simulink model "Elevation_system"  (R2022b)
settings: Solver=VariableStepAuto  StartTime=0.0  StopTime=10  RelTol=1e-4
undefined symbols (not defined in the file): C_pi_pod_elev, C_pi_pod_elev_Kp, gain_notch_pod_elev_tf, k_egun_inv_plant, k_feed_gun_elev, linear_egun_inv_plant, linear_feed_forward_GUN_elev_dist
libraries: slpidlib x2, simulink x1
settings Model: Creator=ohadformanair  LastModifiedBy=ohadformanair
settings SolverCC: ZeroCrossAlgorithm=Adaptive
settings DebuggingCC: MaskedZcDiagnostic=none  IgnoredZcDiagnostic=none
settings ModelReferenceCC: EnableRefExpFcnMdlSchedulingChecks=on

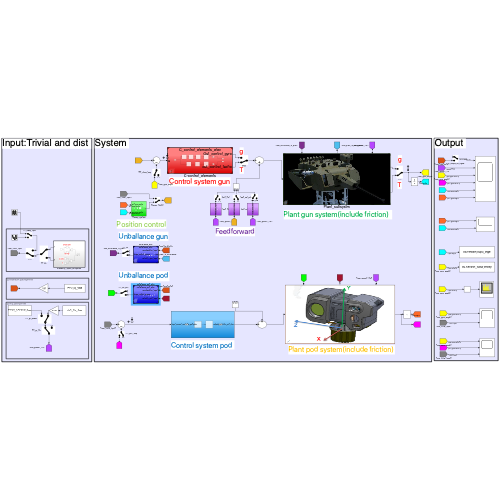
[thumbnail: Simulink's stored preview of the top-level diagram]
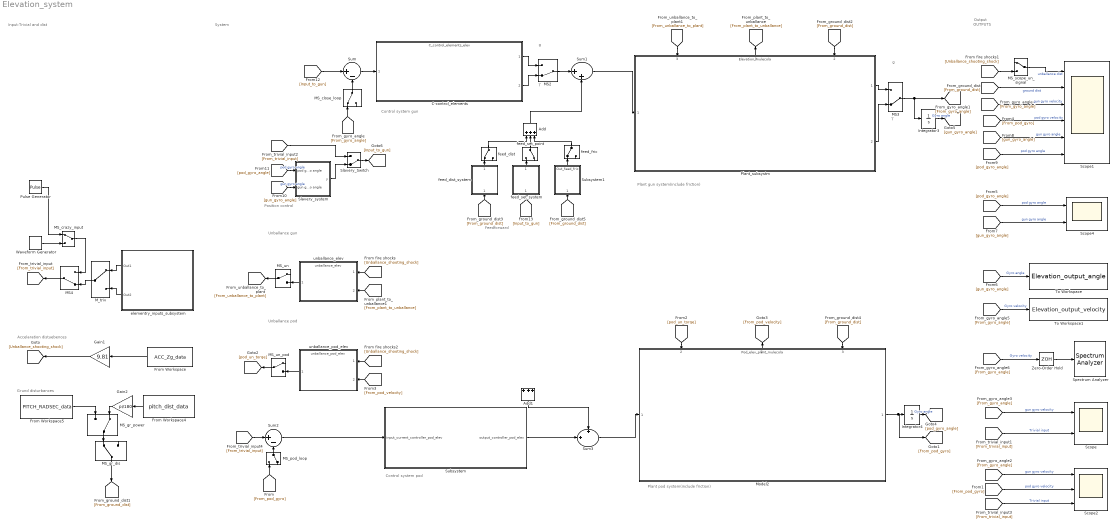
== system Elevation_system ==
  note: Input:Trivial and dist
  note: Control system gun
  note: Accelaration distuebences
  note: Grund disturbances
  note: OUTPUTS
  note: T
  note: T
  note: g
  note: g
  note: Plant gun system(include friction)
  note: Unballance gun
  note: System
  note: Output
  note: Feedforward
  note: Plant pod system(include friction)
  note: Control system pod
  note: Unballance pod
  note: Position control
  Add : Sum  Inputs=+++
  Add1 : Sum  Inputs=+++
  C-control_elements : ModelReference  ModelNameDialog=C_control_elements_elev  SimulationMode=Normal  ModelReferenceVersion=2.0
  From Workspace : FromWorkspace  VariableName=ACC_Zg_data  SampleTime=-1
  From Workspace4 : FromWorkspace  VariableName=pitch_dist_data  SampleTime=-1
  From Workspace5 : FromWorkspace  VariableName=PITCH_RADSEC_data  SampleTime=-1
  Gain1 : Gain  Gain=9.81
  Gain2 : Gain  Gain=pi/180
  Integrator3 : Integrator
  Integrator4 : Integrator
  MS2 : ManualSwitch  CurrentSetting=0
  MS3 : ManualSwitch  CurrentSetting=0
  MS4 : ManualSwitch  CurrentSetting=0
  MS_close_loop : ManualSwitch
  MS_crazy_input : ManualSwitch
  MS_gr_dis : ManualSwitch
  MS_gr_power : ManualSwitch  CurrentSetting=0
  MS_pod_loop : ManualSwitch  CurrentSetting=0
  MS_scope_un_signal : ManualSwitch
  MS_un : ManualSwitch
  MS_un_pod : ManualSwitch
  M_triv : ManualSwitch
  Model2 : ModelReference  ModelNameDialog=Pod_elev_plant_mulecola  SimulationMode=Normal  ModelReferenceVersion=1.13
      settings: PortSchema="{\"entries\":[{\"content\":{\"sides\":[{\"content\":{\"connectorIds\":[\"In1\"]},\"type\":\"ConnectorPlacement.EquallySpacedRectSide\",\"uuid\":\"9e025463-df89-4145-8e3a-d977ce9d23dd\"},{\"content\":{\"connectorIds\":[\"Out1\"],\"side\":\"RIGHT\"},\"type\":\"ConnectorPlacement.EquallySpacedRectSide\",\"uuid\":\"8c795400-902a-445d-a152-b91382759f27\"},{\"content\":{\"connectorIds\":[\"In2\",\"Out2\",\"In3\"],\"side\":\"TOP\"},\"type\":\"ConnectorPlacement.EquallySpacedRectSide\",\"uuid\":\"4797fa26-c9ab-404f-8ecb-3633ee4e5d95\"}]},\"type\":\"ConnectorPlacement.EquallySpacedConnector\",\"uuid\":\"8bb34f86-ba6d-4f3e-a062-415220e2f7a6\"}],\"packageUris\":[\"http://schema.mathworks.com/mf0/Connector/R2020b\"],\"version\":\"1.0\"}"
      mask Display: image('/Users/ohadformanair/Desktop/צילום מסך 2022-12-07 ב-4.14.47.png'); % Use "Edit Image" on toolstrip to change.
  Plant_subsystm : ModelReference  ModelNameDialog=Elevation_mulecola.slx  SimulationMode=Normal  ModelReferenceVersion=2.22
      settings: PortSchema="{\"entries\":[{\"content\":{\"sides\":[{\"content\":{\"connectorIds\":[\"In1\"]},\"type\":\"ConnectorPlacement.EquallySpacedRectSide\",\"uuid\":\"5c3be150-06c1-4b04-81d4-c89054a50b58\"},{\"content\":{\"connectorIds\":[\"Out1\",\"Out2\"],\"side\":\"RIGHT\"},\"type\":\"ConnectorPlacement.EquallySpacedRectSide\",\"uuid\":\"5dfcaa34-ef70-477d-9189-6856ebc4bbcf\"},{\"content\":{\"connectorIds\":[\"In3\",\"Out3\",\"In2\"],\"side\":\"TOP\"},\"type\":\"ConnectorPlacement.EquallySpacedRectSide\",\"uuid\":\"06d3d264-a507-4be0-8bff-1d5586be5fcb\"},{\"content\":{\"connectorIds\":[],\"side\":\"BOTTOM\"},\"type\":\"ConnectorPlacement.EquallySpacedRectSide\",\"uuid\":\"978608b5-cbbf-4f72-8870-46e3c0d8a99d\"}]},\"type\":\"ConnectorPlacement.EquallySpacedConnector\",\"uuid\":\"1f4e30e1-d134-49fc-8bd6-0842cd83f06c\"}],\"packageUris\":[\"http://schema.mathworks.com/mf0/Connector/R2020b\"],\"version\":\"1.0\"}"
      mask Display: image('/Users/ohadformanair/Desktop/צילום מסך 2022-12-07 ב-4.16.46.png'); % Use "Edit Image" on toolstrip to change.
  Pulse Generator : DiscretePulseGenerator  PulseType=Time based  Period=1  PulseWidth=50
  Scope : Scope  NumInputPorts=2
  Scope1 : Scope  NumInputPorts=6
  Scope2 : Scope  NumInputPorts=3
  Scope4 : Scope  NumInputPorts=2
  Slavery_Switch : ManualSwitch  CurrentSetting=0
  Slavery_system : Subsystem
  Spectrum Analyzer : SpectrumAnalyzer
  Subsystem : Subsystem
  Subsystem1 : Subsystem
  Sum : Sum  Inputs=|+-
  Sum1 : Sum  Inputs=|++
  Sum2 : Sum  Inputs=|+-
  Sum3 : Sum  Inputs=+|+||
  To Workspace : ToWorkspace  VariableName=Elevation_output_angle  SaveFormat=Timeseries  SampleTime=-1
  To Workspace1 : ToWorkspace  VariableName=Elevation_output_velocity  SaveFormat=Timeseries  SampleTime=-1
  Waveform Generator : simulink/Sources/Waveform Generator  OutMin=[]  OutMax=[]  OutDataTypeStr=double  SelectedSignal=1  Signals=sin(sawtooth(1,2,0),1,2)+Square(1,2,0,50)#Square(1,2,0,50)  BlockNames=MultiportSwitch_bb3116ca3c8c4cb#MultiportSwitch_6d83ebdfd0d2480  SampleTime=0.01
  Zero-Order Hold : ZeroOrderHold  SampleTime=0.001
  elementry_inputs_subsystem : Subsystem  TreatAsAtomicUnit=on
  feed_dist : ManualSwitch
  feed_dist_system : Subsystem
  feed_fric : ManualSwitch
  feed_set_point : ManualSwitch  CurrentSetting=0
  feed_set_system : Subsystem
  unballance_elev : ModelReference  ModelNameDialog=unballance_elev.slx  SimulationMode=Normal  ModelReferenceVersion=1.10
  unballance_pod_elev : ModelReference  ModelNameDialog=unballance_pod_elev.slx  SimulationMode=Normal  ModelReferenceVersion=1.12
  wires:
  MS_close_loop/1 -> Sum/2
  Plant_subsystm/2 -> MS3/2
  M_triv/1 -> MS4/2
  From Workspace5/1 -> MS_gr_power/1
  MS_gr_power/1 -> MS_gr_dis/1
  [gun_gyro_angle] -> To Workspace/1  "Gyro angle"
  From Workspace4/1 -> Gain2/1
  Gain2/1 -> MS_gr_power/2
  C-control_elements/2 -> MS2/2
  elementry_inputs_subsystem/1(Out1) -> M_triv/1
  elementry_inputs_subsystem/2(Out2) -> M_triv/2
  unballance_elev/1 -> MS_un/2
  Gain1/1 -> [Unballance_shooting_shock]
  C-control_elements/1 -> MS2/1
  Plant_subsystm/1 -> MS3/1
  From Workspace/1 -> Gain1/1
  Sum/1 -> C-control_elements/1
  Zero-Order Hold/1 -> Spectrum Analyzer/1
  MS_scope_un_signal/1 -> Scope1/1  "unballance dist"
  MS2/1 -> Sum1/1
  [Unballance_shooting_shock] -> unballance_elev/1
  [Unballance_shooting_shock] -> MS_scope_un_signal/2
  MS_gr_dis/1 -> [From_ground_dist]
  [From_ground_dist] -> Plant_subsystm/2
  MS3/1 -> [From_gyro_angle], Integrator3/1
  [From_gyro_angle] -> MS_close_loop/1
  [From_trivial_input] -> Slavery_Switch/1
  MS4/1 -> [From_trivial_input]
  Plant_subsystm/3 -> [From_plant_to_unballance]
  [From_plant_to_unballance] -> unballance_elev/2
  MS_un/1 -> [From_unballance_to_plant]
  [From_unballance_to_plant] -> Plant_subsystm/3
  [From_ground_dist] -> Scope1/2  "ground dist"
  Sum1/1 -> Plant_subsystm/1
  Sum2/1 -> Subsystem/1(input_current_controller_pod_elev)
  [From_trivial_input] -> Sum2/1
  MS_pod_loop/1 -> Sum2/2
  Model2/1 -> [From_pod_gyro], Integrator4/1
  Add/1 -> Sum1/2
  feed_dist/1 -> Add/1
  feed_set_point/1 -> Add/2
  [From_ground_dist] -> feed_dist_system/1(feed_dist_input)
  feed_dist_system/1(feed_dist_output) -> feed_dist/1
  feed_set_system/1(feed_set_output) -> feed_set_point/1
  [Input_to_gun] -> feed_set_system/1(feed_set_input)
  [From_trivial_input] -> Scope/2  "Trivial input"
  MS_crazy_input/1 -> MS4/1
  Waveform Generator/1 -> MS_crazy_input/2
  [From_pod_gyro] -> MS_pod_loop/1
  [From_pod_gyro] -> Scope2/2  "pod gyro velocity"
  [From_trivial_input] -> Scope2/3  "Trivial input"
  [From_pod_velocity] -> unballance_pod_elev/2
  Model2/2 -> [From_pod_velocity]
  [Unballance_shooting_shock] -> unballance_pod_elev/1
  unballance_pod_elev/1 -> MS_un_pod/2
  MS_un_pod/1 -> [pod_un_torqe]
  [pod_un_torqe] -> Model2/2
  [From_ground_dist] -> Model2/3
  Subsystem/1(output_controller_pod_elev) -> Sum3/2
  Sum3/1 -> Model2/1
  [From_pod_gyro] -> Scope1/4  "pod gyro velocity"
  [From_gyro_angle] -> Scope2/1  "gun gyro velocity"
  feed_fric/1 -> Add/3
  [From_ground_dist] -> Subsystem1/1(In_dist_velocity)
  Subsystem1/1(Out_feed_fric) -> feed_fric/1
  Integrator3/1 -> [gun_gyro_angle]  "Gyro angle"
  Integrator4/1 -> [pod_gyro_angle]  "Gyro angle"
  [pod_gyro_angle] -> Scope4/1  "pod gyro angle"
  [gun_gyro_angle] -> Scope4/2  "gun gyro angle"
  [gun_gyro_angle] -> Scope1/5  "gun gyro angle"
  [From_gyro_angle] -> Scope/1  "gun gyro velocity"
  [From_gyro_angle] -> To Workspace1/1  "Gyro velocity"
  [From_gyro_angle] -> Scope1/3  "gun gyro velocity"
  [pod_gyro_angle] -> Scope1/6  "pod gyro angle"
  [From_gyro_angle] -> Zero-Order Hold/1  "Gyro velocity"
  Add1/1 -> Sum3/1
  Slavery_Switch/1 -> [Input_to_gun]
  [pod_gyro_angle] -> Slavery_system/1(pod gyro angle)  "pod gyro angle"
  [gun_gyro_angle] -> Slavery_system/2(gun gyro angle)  "gun gyro angle"
  Slavery_system/1(y) -> Slavery_Switch/2
  [Input_to_gun] -> Sum/1
  Pulse Generator/1 -> MS_crazy_input/1

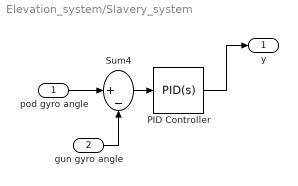
== system Elevation_system/Slavery_system ==
  pod gyro angle : Inport
  gun gyro angle : Inport  Port=2
  PID Controller : slpidlib/PID Controller  Controller=PID  Form=Parallel  TimeDomain=Continuous-time  UseExternalTs=off  SampleTime=-1  IntegratorMethod=Forward Euler  FilterMethod=Forward Euler  ControllerParametersSource=internal  P=28.4604839223426+30  I=9.47112032466826  UseKiTs=off  D=0.287192930745774  N=4361.00624343209  UseFilter=on  TunerSelectOption=Transfer Function Based (PID Tuner App)  InitialConditionSource=internal  InitialConditionForIntegrator=0  InitialConditionForFilter=0  DifferentiatorICPrevScaledInput=0  ExternalReset=none  TrackingMode=off  Kt=1  LimitOutput=off  SatLimitsSource=internal  UpperSaturationLimit=inf  LowerSaturationLimit=-inf  LinearizeAsGain=on  AntiWindupMode=none  Kb=1  LimitIntegrator=off  UpperIntegratorSaturationLimit=inf  LowerIntegratorSaturationLimit=-inf  POutMin=[]  POutMax=[]  IOutMin=[]  IOutMax=[]  DOutMin=[]  DOutMax=[]  NOutMin=[]  NOutMax=[]  SumOutMin=[]  SumOutMax=[]  SaturationOutMin=[]  SaturationOutMax=[]  PParamMin=[]  PParamMax=[]  IParamMin=[]  IParamMax=[]  DParamMin=[]  DParamMax=[]  NParamMin=[]  NParamMax=[]  KbParamMin=[]  KbParamMax=[]  KtParamMin=[]  KtParamMax=[]  KbOutMin=[]  KbOutMax=[]  KtOutMin=[]  KtOutMax=[]  IntegratorOutMin=[]  IntegratorOutMax=[]  FilterOutMin=[]  FilterOutMax=[]  SumI1OutMin=[]  SumI1OutMax=[]  SumI2OutMin=[]  SumI2OutMax=[]  SumI3OutMin=[]  SumI3OutMax=[]  SumI4OutMin=[]  SumI4OutMax=[]  SumDOutMin=[]  SumDOutMax=[]  DifferentiatorOutMin=[]  DifferentiatorOutMax=[]  FilterDiffOutCoefMin=[]  FilterDiffOutCoefMax=[]  ReciprocalOutMin=[]  ReciprocalOutMax=[]  SumDenOutMin=[]  SumDenOutMax=[]  SumNumOutMin=[]  SumNumOutMax=[]  DivideOutMin=[]  DivideOutMax=[]  UdiffTsProdOutMin=[]  UdiffTsProdOutMax=[]  NTsProdOutMin=[]  NTsProdOutMax=[]  UintegralTsProdOutMin=[]  UintegralTsProdOutMax=[]  UngainTsProdOutMin=[]  UngainTsProdOutMax=[]  ClampingZeroOutDataTypeStr=Inherit: Inherit via back propagation  ClampingZeroOutMin=[]  ClampingZeroOutMax=[]  FilterDenConstantOutDataTypeStr=Inherit: Inherit via back propagation  FilterDenConstantOutMin=[]  FilterDenConstantOutMax=[]  PCopyOutDataTypeStr=Inherit: Inherit via back propagation  PCopyOutMin=[]  PCopyOutMax=[]  NCopyOutDataTypeStr=Inherit: Inherit via back propagation  NCopyOutMin=[]  NCopyOutMax=[]  IntegratorContinuousStateAttributes=''  IntegratorStateMustResolveToSignalObject=off  IntegratorRTWStateStorageClass=Auto  FilterContinuousStateAttributes=''  FilterStateMustResolveToSignalObject=off  FilterRTWStateStorageClass=Auto  ParallelPVariant=InternalParameters  IdealPVariant=Disabled  IVariant=InternalParameters  DVariant=InternalParameters  IntegratorVariant=Continuous  SatVariant=Disabled  AWVariant=Passthrough  PCopyVariant=Disabled  TRVariant=Disabled  FdbkBlocksVariant=Forward  IdealPFdbkVariant=Disabled  SatFdbkVariant=Disabled  DerivativeFilterVariant=ContFilter  NVariant=InternalParameters  NCopyVariant=Disabled  FilterICVariant=InternalICsFilter  IntegratorICVariant=InternalICs  ExternalResetVariant=Disabled  TRSumVariant=Passthrough  SumFdbkVariant=Disabled  SumVariant=Sum_PID  TsampFilterVariant=InternalTs  TsampNgainVariant=Passthrough  TsampIntegralVariant=Passthrough  ExternalSaturationOutDataTypeStr=Inherit: Same as second input
  Sum4 : Sum  Inputs=|+-
  y : Outport
  wires:
  pod gyro angle/1 -> Sum4/1
  PID Controller/1 -> y/1
  gun gyro angle/1 -> Sum4/2
  Sum4/1 -> PID Controller/1

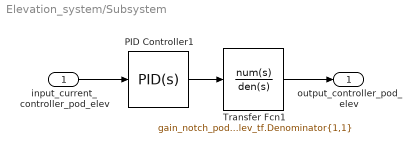
== system Elevation_system/Subsystem ==
  input_current_controller_pod_elev : Inport
  PID Controller1 : slpidlib/PID Controller  Controller=PID  Form=Parallel  TimeDomain=Continuous-time  UseExternalTs=off  SampleTime=-1  IntegratorMethod=Forward Euler  FilterMethod=Forward Euler  ControllerParametersSource=internal  P=C_pi_pod_elev_Kp  I=C_pi_pod_elev.Ki  UseKiTs=off  D=0  N=0  UseFilter=on  TunerSelectOption=Transfer Function Based (PID Tuner App)  InitialConditionSource=internal  InitialConditionForIntegrator=0  InitialConditionForFilter=0  DifferentiatorICPrevScaledInput=0  ExternalReset=none  TrackingMode=off  Kt=1  LimitOutput=off  SatLimitsSource=internal  UpperSaturationLimit=inf  LowerSaturationLimit=-inf  LinearizeAsGain=on  AntiWindupMode=none  Kb=1  LimitIntegrator=off  UpperIntegratorSaturationLimit=inf  LowerIntegratorSaturationLimit=-inf  POutMin=[]  POutMax=[]  IOutMin=[]  IOutMax=[]  DOutMin=[]  DOutMax=[]  NOutMin=[]  NOutMax=[]  SumOutMin=[]  SumOutMax=[]  SaturationOutMin=[]  SaturationOutMax=[]  PParamMin=[]  PParamMax=[]  IParamMin=[]  IParamMax=[]  DParamMin=[]  DParamMax=[]  NParamMin=[]  NParamMax=[]  KbParamMin=[]  KbParamMax=[]  KtParamMin=[]  KtParamMax=[]  KbOutMin=[]  KbOutMax=[]  KtOutMin=[]  KtOutMax=[]  IntegratorOutMin=[]  IntegratorOutMax=[]  FilterOutMin=[]  FilterOutMax=[]  SumI1OutMin=[]  SumI1OutMax=[]  SumI2OutMin=[]  SumI2OutMax=[]  SumI3OutMin=[]  SumI3OutMax=[]  SumI4OutMin=[]  SumI4OutMax=[]  SumDOutMin=[]  SumDOutMax=[]  DifferentiatorOutMin=[]  DifferentiatorOutMax=[]  FilterDiffOutCoefMin=[]  FilterDiffOutCoefMax=[]  ReciprocalOutMin=[]  ReciprocalOutMax=[]  SumDenOutMin=[]  SumDenOutMax=[]  SumNumOutMin=[]  SumNumOutMax=[]  DivideOutMin=[]  DivideOutMax=[]  UdiffTsProdOutMin=[]  UdiffTsProdOutMax=[]  NTsProdOutMin=[]  NTsProdOutMax=[]  UintegralTsProdOutMin=[]  UintegralTsProdOutMax=[]  UngainTsProdOutMin=[]  UngainTsProdOutMax=[]  ClampingZeroOutDataTypeStr=Inherit: Inherit via back propagation  ClampingZeroOutMin=[]  ClampingZeroOutMax=[]  FilterDenConstantOutDataTypeStr=Inherit: Inherit via back propagation  FilterDenConstantOutMin=[]  FilterDenConstantOutMax=[]  PCopyOutDataTypeStr=Inherit: Inherit via back propagation  PCopyOutMin=[]  PCopyOutMax=[]  NCopyOutDataTypeStr=Inherit: Inherit via back propagation  NCopyOutMin=[]  NCopyOutMax=[]  IntegratorContinuousStateAttributes=''  IntegratorStateMustResolveToSignalObject=off  IntegratorRTWStateStorageClass=Auto  FilterContinuousStateAttributes=''  FilterStateMustResolveToSignalObject=off  FilterRTWStateStorageClass=Auto  ParallelPVariant=InternalParameters  IdealPVariant=Disabled  IVariant=InternalParameters  DVariant=InternalParameters  IntegratorVariant=Continuous  SatVariant=Disabled  AWVariant=Passthrough  PCopyVariant=Disabled  TRVariant=Disabled  FdbkBlocksVariant=Forward  IdealPFdbkVariant=Disabled  SatFdbkVariant=Disabled  DerivativeFilterVariant=ContFilter  NVariant=InternalParameters  NCopyVariant=Disabled  FilterICVariant=InternalICsFilter  IntegratorICVariant=InternalICs  ExternalResetVariant=Disabled  TRSumVariant=Passthrough  SumFdbkVariant=Disabled  SumVariant=Sum_PID  TsampFilterVariant=InternalTs  TsampNgainVariant=Passthrough  TsampIntegralVariant=Passthrough  ExternalSaturationOutDataTypeStr=Inherit: Same as second input
  Transfer Fcn1 : TransferFcn  Numerator=gain_notch_pod_elev_tf.Numerator{1,1}  Denominator=gain_notch_pod_elev_tf.Denominator{1,1}
  output_controller_pod_elev : Outport
  wires:
  input_current_controller_pod_elev/1 -> PID Controller1/1
  Transfer Fcn1/1 -> output_controller_pod_elev/1
  PID Controller1/1 -> Transfer Fcn1/1

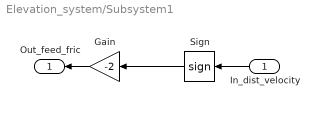
== system Elevation_system/Subsystem1 ==
  In_dist_velocity : Inport
  Gain : Gain  Gain=-2
  Sign : Signum
  Out_feed_fric : Outport
  wires:
  Gain/1 -> Out_feed_fric/1
  In_dist_velocity/1 -> Sign/1
  Sign/1 -> Gain/1

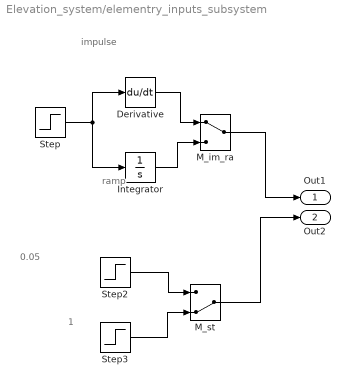
== system Elevation_system/elementry_inputs_subsystem ==
  note: impulse
  note: ramp
  note: 0.05
  note: 1
  Derivative : Derivative
  Integrator : Integrator
  M_im_ra : ManualSwitch
  M_st : ManualSwitch  CurrentSetting=0
  Step : Step  SampleTime=0
  Step2 : Step  After=0.05  SampleTime=0
  Step3 : Step  SampleTime=0
  Out1 : Outport
  Out2 : Outport  Port=2
  wires:
  M_st/1 -> Out2/1
  Step3/1 -> M_st/2
  Derivative/1 -> M_im_ra/1
  M_im_ra/1 -> Out1/1
  Step/1 -> Integrator/1, Derivative/1
  Step2/1 -> M_st/1
  Integrator/1 -> M_im_ra/2

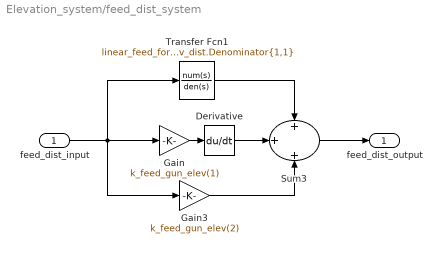
== system Elevation_system/feed_dist_system ==
  feed_dist_input : Inport
  Derivative : Derivative
  Gain : Gain  Gain=k_feed_gun_elev(1)
  Gain3 : Gain  Gain=k_feed_gun_elev(2)
  Sum3 : Sum  Inputs=+|+|+
  Transfer Fcn1 : TransferFcn  Numerator=linear_feed_forward_GUN_elev_dist.Numerator{1,1}  Denominator=linear_feed_forward_GUN_elev_dist.Denominator{1,1}
  feed_dist_output : Outport
  wires:
  Sum3/1 -> feed_dist_output/1
  Derivative/1 -> Sum3/2
  feed_dist_input/1 -> Gain/1, Gain3/1, Transfer Fcn1/1
  Transfer Fcn1/1 -> Sum3/1
  Gain/1 -> Derivative/1
  Gain3/1 -> Sum3/3

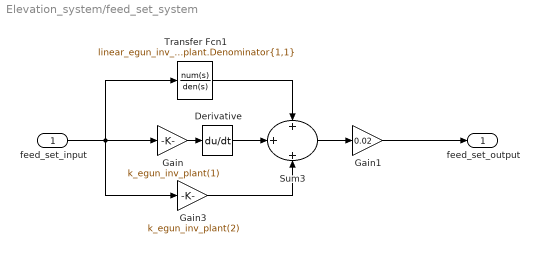
== system Elevation_system/feed_set_system ==
  feed_set_input : Inport
  Derivative : Derivative
  Gain : Gain  Gain=k_egun_inv_plant(1)
  Gain1 : Gain  Gain=0.02
  Gain3 : Gain  Gain=k_egun_inv_plant(2)
  Sum3 : Sum  Inputs=+|+|+
  Transfer Fcn1 : TransferFcn  Numerator=linear_egun_inv_plant.Numerator{1,1}  Denominator=linear_egun_inv_plant.Denominator{1,1}
  feed_set_output : Outport
  wires:
  Derivative/1 -> Sum3/2
  feed_set_input/1 -> Gain/1, Gain3/1, Transfer Fcn1/1
  Transfer Fcn1/1 -> Sum3/1
  Gain/1 -> Derivative/1
  Gain3/1 -> Sum3/3
  Sum3/1 -> Gain1/1
  Gain1/1 -> feed_set_output/1
